simulink model "actividad1_22simulink"  (R2021a)
settings: Solver=ode1  StartTime=0.0  StopTime=3  FixedStep=0.001  RelTol=1e-3
libraries: simulink_need_slupdate x6
settings Model: Creator=Agus  LastModifiedBy=Agus

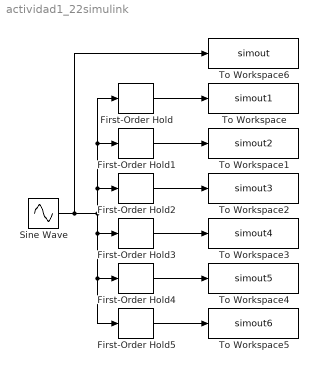
== system actividad1_22simulink ==
  First-Order Hold : simulink_need_slupdate/First-Order Hold  DisableCoverage=on  Ts=0.75
      settings: SourceProductBaseCode=SL
  First-Order Hold1 : simulink_need_slupdate/First-Order Hold  DisableCoverage=on  Ts=0.5
      settings: SourceProductBaseCode=SL
  First-Order Hold2 : simulink_need_slupdate/First-Order Hold  DisableCoverage=on  Ts=0.2
      settings: SourceProductBaseCode=SL
  First-Order Hold3 : simulink_need_slupdate/First-Order Hold  DisableCoverage=on  Ts=0.1
      settings: SourceProductBaseCode=SL
  First-Order Hold4 : simulink_need_slupdate/First-Order Hold  DisableCoverage=on  Ts=0.05
      settings: SourceProductBaseCode=SL
  First-Order Hold5 : simulink_need_slupdate/First-Order Hold  DisableCoverage=on  Ts=0.01
      settings: SourceProductBaseCode=SL
  Sine Wave : Sin  Frequency=2*pi  SampleTime=0
  To Workspace : ToWorkspace  VariableName=simout1  SaveFormat=Timeseries  SampleTime=-1
  To Workspace1 : ToWorkspace  VariableName=simout2  SaveFormat=Timeseries  SampleTime=-1
  To Workspace2 : ToWorkspace  VariableName=simout3  SaveFormat=Timeseries  SampleTime=-1
  To Workspace3 : ToWorkspace  VariableName=simout4  SaveFormat=Timeseries  SampleTime=-1
  To Workspace4 : ToWorkspace  VariableName=simout5  SaveFormat=Timeseries  SampleTime=-1
  To Workspace5 : ToWorkspace  VariableName=simout6  SaveFormat=Timeseries  SampleTime=-1
  To Workspace6 : ToWorkspace  VariableName=simout  SaveFormat=Timeseries  SampleTime=-1
  wires:
  First-Order Hold1/1 -> To Workspace1/1
  First-Order Hold4/1 -> To Workspace4/1
  First-Order Hold2/1 -> To Workspace2/1
  First-Order Hold3/1 -> To Workspace3/1
  Sine Wave/1 -> To Workspace6/1, First-Order Hold2/1, First-Order Hold1/1, First-Order Hold/1, First-Order Hold3/1, First-Order Hold5/1, First-Order Hold4/1
  First-Order Hold/1 -> To Workspace/1
  First-Order Hold5/1 -> To Workspace5/1
